simulink model "lif_neuron"  (Simulink 8.3)
settings: Solver=ode45  StartTime=0.0  StopTime=2  RelTol=1e-3
values from neighbouring files (symbols this model uses):
  current_gain = 20    [test_lif_neuron.m]    (also in test_stdp_synapse.m = 10)
  neu_decay = 5    [test_lif_neuron.m]    (also in test_stdp_synapse.m = 0.5)
  neu_th = 0.02    [test_lif_neuron.m]    (also in test_stdp_synapse.m)
  raf_delay = 0.02    [test_lif_neuron.m]
  spike_period = [0.015]    [test_lif_neuron.m]    (also in test_stdp_synapse.m = (4 + 0.2*t_extra)/3*0.03)
undefined symbols (not defined in the file): pulse_width
libraries: simulink x1
settings Model: Creator=wjj  LastModifiedBy=wjj
settings DataIOCC: SignalLoggingSaveFormat=Dataset
settings DebuggingCC: UnderspecifiedInitializationDetection=Simplified  StateNameClashWarn=none
settings GRTTargetCC: CombineOutputUpdateFcns=on  GRTInterface=off

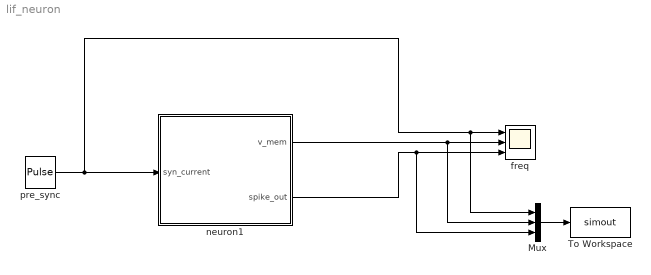
== system lif_neuron ==
  Mux : Mux  Inputs=3
  To Workspace : ToWorkspace  VariableName=simout  SampleTime=5e-4
      settings: Save2DSignal=2-D array (concatenate along first dimension)
  freq : Scope  NumInputPorts=3
      settings: TimeRange=1  YMin=0~0~0  YMax=1.2~0.1~1.2
  neuron1 : Subsystem  mask{neu_th=neu_th, pulse_width=pulse_width, neu_decay=neu_decay, current_gain=current_gain}
      mask prompts: neu_th "Neuron threshold"; pulse_width "Spike pulse width"; current_gain "Current Gain"
      mask DialogControl DescTextVar Prompt: Neuron module receives weighted spikes, and generates neuron spikes.
  pre_sync : DiscretePulseGenerator  PulseType=Time based  Period=spike_period(1)  PulseWidth=0.05/spike_period(1)  PhaseDelay=spike_period(1)/2
  wires:
  pre_sync/1 -> Mux/1, freq/1, neuron1/1(syn_current)
  Mux/1 -> To Workspace/1
  neuron1/1(v_mem) -> Mux/2, freq/2
  neuron1/2(spike_out) -> Mux/3, freq/3

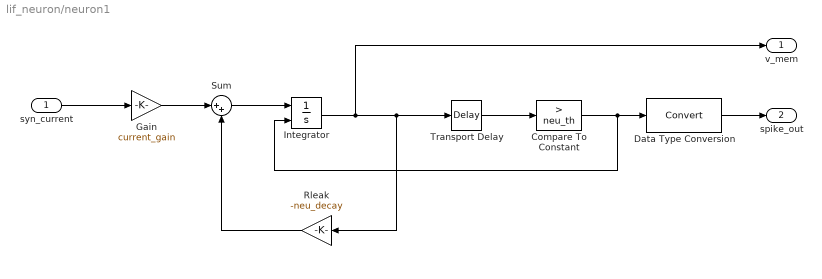
== system lif_neuron/neuron1 ==
  syn_current : Inport
  Compare To Constant : simulink/Logic and Bit Operations/Compare To Constant  relop=>  const=neu_th  OutDataTypeStr=boolean
  Data Type Conversion : DataTypeConversion
  Gain : Gain  Gain=current_gain
  Integrator : Integrator  ExternalReset=rising  LimitOutput=on  LowerSaturationLimit=0
  Rleak : Gain  Gain=-neu_decay
  Sum : Sum  Inputs=|++
  Transport Delay : TransportDelay  DelayTime=raf_delay
  v_mem : Outport
  spike_out : Outport  Port=2
  wires:
  Transport Delay/1 -> Compare To Constant/1
  Compare To Constant/1 -> Data Type Conversion/1, Integrator/2
  Integrator/1 -> Rleak/1, Transport Delay/1, v_mem/1
  Sum/1 -> Integrator/1
  Data Type Conversion/1 -> spike_out/1
  syn_current/1 -> Gain/1
  Gain/1 -> Sum/1
  Rleak/1 -> Sum/2
